simulink model "sgp4_eci_comparison"  (R2018b)
settings: Solver=FixedStepAuto  StartTime=0.0  StopTime=15000  FixedStep=simParams.sample_time_s  RelTol=1e-3
libraries: CDH_command_lib x1, Environment_lib x1, FSW_Lib x1, satelliteDynamics_lib x1
settings Model: Creator=colem  LastModifiedBy=colem

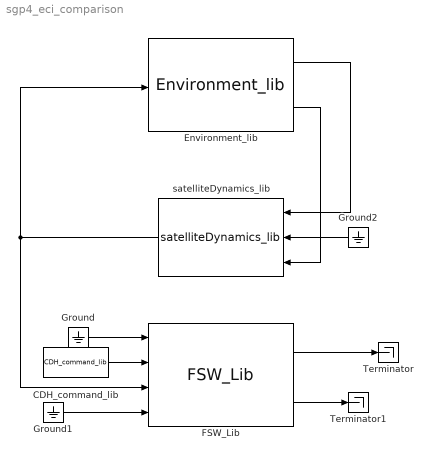
== system sgp4_eci_comparison ==
  CDH_command_lib : CDH_command_lib/CDH_command_lib  SystemSampleTime=-1
  Environment_lib : Environment_lib/Environment_lib  SystemSampleTime=-1
  FSW_Lib : FSW_Lib/FSW_Lib  SystemSampleTime=-1
  Ground : Ground
  Ground1 : Ground
  Ground2 : Ground
  Terminator : Terminator
  Terminator1 : Terminator
  satelliteDynamics_lib : satelliteDynamics_lib/satelliteDynamics_lib  SystemSampleTime=-1
  wires:
  satelliteDynamics_lib/1 -> Environment_lib/1, FSW_Lib/3
  CDH_command_lib/1 -> FSW_Lib/2
  Ground/1 -> FSW_Lib/1
  Ground1/1 -> FSW_Lib/4
  Environment_lib/1 -> satelliteDynamics_lib/1
  Environment_lib/2 -> satelliteDynamics_lib/3
  Ground2/1 -> satelliteDynamics_lib/2
  FSW_Lib/1 -> Terminator/1
  FSW_Lib/2 -> Terminator1/1
